simulink model "AM2"  (Simulink 8.3)
settings: Solver=ode45  StartTime=0.0  StopTime=2  RelTol=1e-3
undefined symbols (not defined in the file): get
libraries: dspspect3 x1, dspsnks4 x1
settings Model: Creator=sesay  LastModifiedBy=maalmasr
settings DataIOCC: SignalLoggingSaveFormat=Dataset  SignalLoggingName=sigsOut
settings OptimizationCC: ExpressionDepthLimit=2147483647
settings DebuggingCC: SaveWithParameterizedLinksMsg=none  SignalResolutionControl=TryResolveAllWithWarning  SolverPrmCheckMsg=none  MultiTaskDSMMsg=warning  MultiTaskCondExecSysMsg=none
settings HardwareCC: TargetUnknown=on
settings RTWCC: IncludeERTFirstTime=on

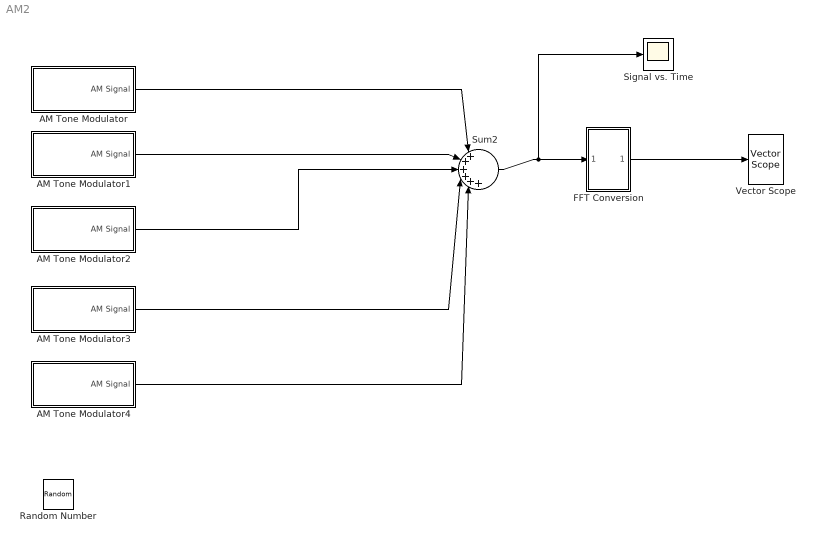
== system AM2 ==
  AM Tone Modulator : Subsystem  mask{Fc=1000, Fm=100, m=0.4}
      mask prompts: Fc "Carrier Frequency"; Fm "Message Frequency"; m "Modulation Index"
  AM Tone Modulator1 : Subsystem  mask{Fc=1000, Fm=200, m=1}
      mask prompts: Fc "Carrier Frequency"; Fm "Message Frequency"; m "Modulation Index"
  AM Tone Modulator2 : Subsystem  mask{Fc=1000, Fm=100, m=0.4}
      mask prompts: Fc "Carrier Frequency"; Fm "Message Frequency"; m "Modulation Index"
  AM Tone Modulator3 : Subsystem  mask{Fc=1000, Fm=200, m=1}
      mask prompts: Fc "Carrier Frequency"; Fm "Message Frequency"; m "Modulation Index"
  AM Tone Modulator4 : Subsystem  mask{Fc=1000, Fm=100, m=0.4}
      mask prompts: Fc "Carrier Frequency"; Fm "Message Frequency"; m "Modulation Index"
  FFT Conversion : Subsystem
  Random Number : RandomNumber  Variance=3  SampleTime=1/8000
  Signal vs. Time : Scope
      settings: TickLabels=on  SampleInput=on  SampleTime=1/8000
  Sum2 : Sum  Inputs=|++++++  SaturateOnIntegerOverflow=on
  Vector Scope : dspsnks4/Vector Scope  ScopeProperties=off  Domain=Frequency  HorizSpan=1  DisplayProperties=off  AxisGrid=on  Memory=off  FrameNumber=on  AxisLegend=off  AxisZoom=off  OpenScopeAtSimStart=on  OpenScopeImmediately=off  FigPos=get(0,'defaultfigureposition')  AxisProperties=on  XUnits=Hertz  XRange=[0...Fs/2]  InheritXIncr=on  XIncr=1  XLabel=Time  XLimit=Auto  XMin=0  XMax=1  XStart=0  YUnits=Magnitude  YLabel=Amplitude  LineProperties=off  XAxisParamsVer=6.9
      settings: YMin=0.000318299870930715  YMax=0.548504340064008
  wires:
  FFT Conversion/1(Out1) -> Vector Scope/1
  Sum2/1 -> FFT Conversion/1(In1), Signal vs. Time/1
  AM Tone Modulator/1(AM Signal) -> Sum2/1
  AM Tone Modulator1/1(AM Signal) -> Sum2/2
  AM Tone Modulator2/1(AM Signal) -> Sum2/3
  AM Tone Modulator3/1(AM Signal) -> Sum2/4
  AM Tone Modulator4/1(AM Signal) -> Sum2/5

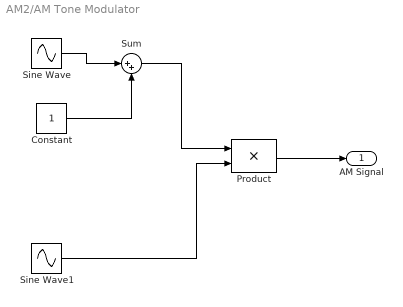
== system AM2/AM Tone Modulator ==
  Constant : Constant
  Product : Product  SaturateOnIntegerOverflow=on  OutDataTypeStr=Inherit: Same as first input
  Sine Wave : Sin  Amplitude=m  Frequency=Fm*2*pi  Phase=pi/2  SampleTime=1/8000
  Sine Wave1 : Sin  Frequency=Fc*2*pi  Phase=pi/2  SampleTime=1/8000
  Sum : Sum  Inputs=|++  SaturateOnIntegerOverflow=on
  AM Signal : Outport
  wires:
  Sine Wave1/1 -> Product/2
  Sine Wave/1 -> Sum/1
  Constant/1 -> Sum/2
  Sum/1 -> Product/1
  Product/1 -> AM Signal/1

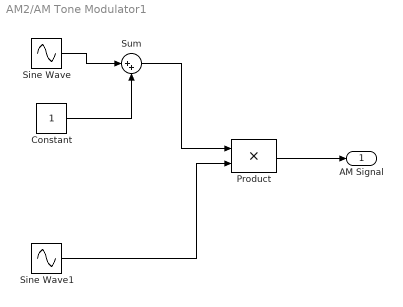
== system AM2/AM Tone Modulator1 ==
  Constant : Constant
  Product : Product  SaturateOnIntegerOverflow=on  OutDataTypeStr=Inherit: Same as first input
  Sine Wave : Sin  Amplitude=m  Frequency=Fm*2*pi  Phase=pi/2  SampleTime=1/8000
  Sine Wave1 : Sin  Frequency=Fc*2*pi  Phase=pi/2  SampleTime=1/8000
  Sum : Sum  Inputs=|++  SaturateOnIntegerOverflow=on
  AM Signal : Outport
  wires:
  Sine Wave1/1 -> Product/2
  Sine Wave/1 -> Sum/1
  Constant/1 -> Sum/2
  Sum/1 -> Product/1
  Product/1 -> AM Signal/1

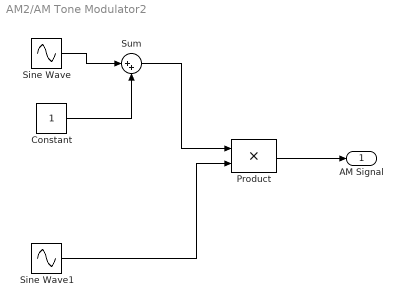
== system AM2/AM Tone Modulator2 ==
  Constant : Constant
  Product : Product  SaturateOnIntegerOverflow=on  OutDataTypeStr=Inherit: Same as first input
  Sine Wave : Sin  Amplitude=m  Frequency=Fm*2*pi  Phase=pi/2  SampleTime=1/8000
  Sine Wave1 : Sin  Frequency=Fc*2*pi  Phase=pi/2  SampleTime=1/8000
  Sum : Sum  Inputs=|++  SaturateOnIntegerOverflow=on
  AM Signal : Outport
  wires:
  Sine Wave1/1 -> Product/2
  Sine Wave/1 -> Sum/1
  Constant/1 -> Sum/2
  Sum/1 -> Product/1
  Product/1 -> AM Signal/1

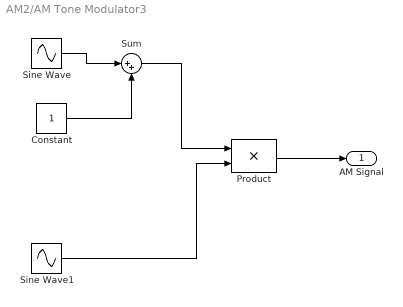
== system AM2/AM Tone Modulator3 ==
  Constant : Constant
  Product : Product  SaturateOnIntegerOverflow=on  OutDataTypeStr=Inherit: Same as first input
  Sine Wave : Sin  Amplitude=m  Frequency=Fm*2*pi  Phase=pi/2  SampleTime=1/8000
  Sine Wave1 : Sin  Frequency=Fc*2*pi  Phase=pi/2  SampleTime=1/8000
  Sum : Sum  Inputs=|++  SaturateOnIntegerOverflow=on
  AM Signal : Outport
  wires:
  Sine Wave1/1 -> Product/2
  Sine Wave/1 -> Sum/1
  Constant/1 -> Sum/2
  Sum/1 -> Product/1
  Product/1 -> AM Signal/1

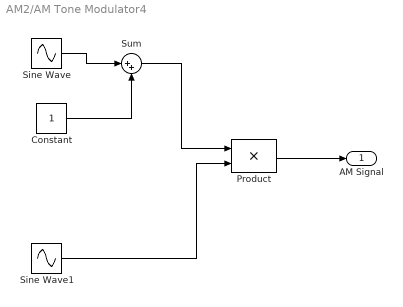
== system AM2/AM Tone Modulator4 ==
  Constant : Constant
  Product : Product  SaturateOnIntegerOverflow=on  OutDataTypeStr=Inherit: Same as first input
  Sine Wave : Sin  Amplitude=m  Frequency=Fm*2*pi  Phase=pi/2  SampleTime=1/8000
  Sine Wave1 : Sin  Frequency=Fc*2*pi  Phase=pi/2  SampleTime=1/8000
  Sum : Sum  Inputs=|++  SaturateOnIntegerOverflow=on
  AM Signal : Outport
  wires:
  Sine Wave1/1 -> Product/2
  Sine Wave/1 -> Sum/1
  Constant/1 -> Sum/2
  Sum/1 -> Product/1
  Product/1 -> AM Signal/1

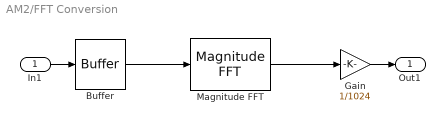
== system AM2/FFT Conversion ==
  In1 : Inport
  Buffer : Buffer  N=1024  TreatMby1Signals=One channel
  Gain : Gain  Gain=1/1024  SaturateOnIntegerOverflow=on  OutDataTypeStr=Inherit: Same as input  ParamDataTypeStr=Inherit: Same as input
  Magnitude FFT : dspspect3/Magnitude FFT  mag_or_magsq=Magnitude  FFTImplementation=Auto  fftLenInherit=on  fftsize=256  WrapInput=on
  Out1 : Outport
  wires:
  Buffer/1 -> Magnitude FFT/1
  Magnitude FFT/1 -> Gain/1
  In1/1 -> Buffer/1
  Gain/1 -> Out1/1
